simulink model "w2project2"  (R2020b)
settings: Solver=VariableStepAuto  StartTime=0.0  StopTime=10.0  RelTol=1e-3
model workspace (MAT data in the model file):
  Ie = 1
  Iv = 5
  R = 1
  be = 2
  bv = 1
  uk = 1
  us = 1.5
settings Model: Creator=rutvi  LastModifiedBy=rutvi

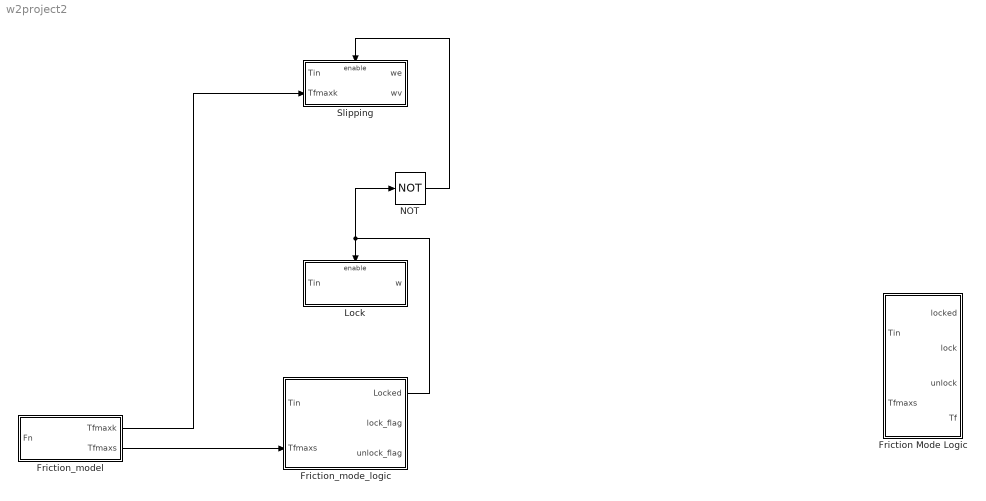
== system w2project2 ==
  Friction Mode Logic : Subsystem
      mask Display: plot([-3 1 1 3 -1 -1],[-1 -1 1 1 1 -1],-4,-5,4,5)
  Friction_mode_logic : Subsystem
  Friction_model : Subsystem
  Lock : Subsystem
  NOT : Logic  Operator=NOT  IconShape=distinctive  AllPortsSameDT=off  OutDataTypeStr=boolean
  Slipping : Subsystem
  wires:
  Friction_model/2(Tfmaxs) -> Friction_mode_logic/2(Tfmaxs)
  Friction_model/1(Tfmaxk) -> Slipping/2(Tfmaxk)
  Friction_mode_logic/1(Locked) -> NOT/1, Lock/Enable
  NOT/1 -> Slipping/Enable

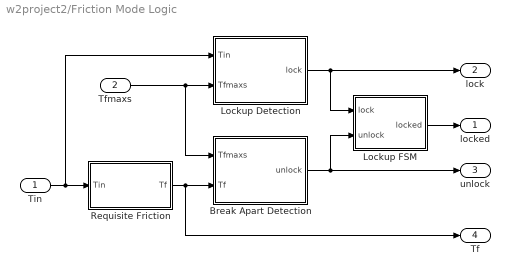
== system w2project2/Friction Mode Logic ==
  Tin : Inport
  Tfmaxs : Inport  Port=2
  Break Apart Detection : Subsystem
  Lockup Detection : Subsystem
  Lockup FSM : Subsystem
  Requisite Friction : Subsystem
  locked : Outport  InitialOutput=0  VectorParamsAs1DForOutWhenUnconnected=off
  lock : Outport  Port=2  InitialOutput=0  VectorParamsAs1DForOutWhenUnconnected=off
  unlock : Outport  Port=3  InitialOutput=0  VectorParamsAs1DForOutWhenUnconnected=off
  Tf : Outport  Port=4  InitialOutput=0  VectorParamsAs1DForOutWhenUnconnected=off
  wires:
  Tin/1 -> Lockup Detection/1(Tin), Requisite Friction/1(Tin)
  Tfmaxs/1 -> Lockup Detection/2(Tfmaxs), Break Apart Detection/1(Tfmaxs)
  Requisite Friction/1(Tf) -> Break Apart Detection/2(Tf), Tf/1
  Break Apart Detection/1(unlock) -> Lockup FSM/2(unlock), unlock/1
  Lockup Detection/1(lock) -> Lockup FSM/1(lock), lock/1
  Lockup FSM/1(locked) -> locked/1

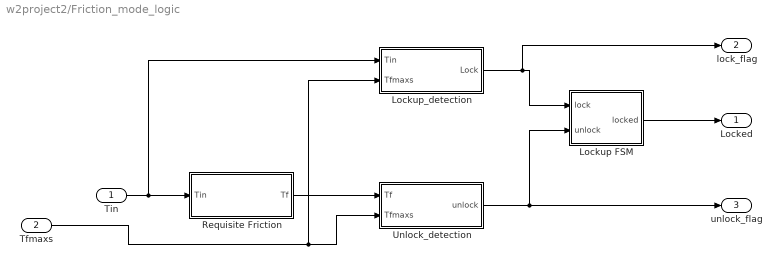
== system w2project2/Friction_mode_logic ==
  Tin : Inport
  Tfmaxs : Inport  Port=2
  Lockup FSM : Subsystem
  Lockup_detection : Subsystem
  Requisite Friction : Subsystem
  Unlock_detection : Subsystem
  Locked : Outport
  lock_flag : Outport  Port=2
  unlock_flag : Outport  Port=3
  wires:
  Lockup_detection/1(Lock) -> lock_flag/1, Lockup FSM/1(lock)
  Unlock_detection/1(unlock) -> unlock_flag/1, Lockup FSM/2(unlock)
  Lockup FSM/1(locked) -> Locked/1
  Requisite Friction/1(Tf) -> Unlock_detection/1(Tf)
  Tfmaxs/1 -> Lockup_detection/2(Tfmaxs), Unlock_detection/2(Tfmaxs)
  Tin/1 -> Lockup_detection/1(Tin), Requisite Friction/1(Tin)

== system w2project2/Friction_model ==
  Fn : Inport
  Gain : Gain  Gain=0.66*R*us
  Gain1 : Gain  Gain=0.66*R*uk
  Tfmaxk : Outport
  Tfmaxs : Outport  Port=2
  wires:
  Gain1/1 -> Tfmaxk/1
  Gain/1 -> Tfmaxs/1
  Fn/1 -> Gain1/1, Gain/1

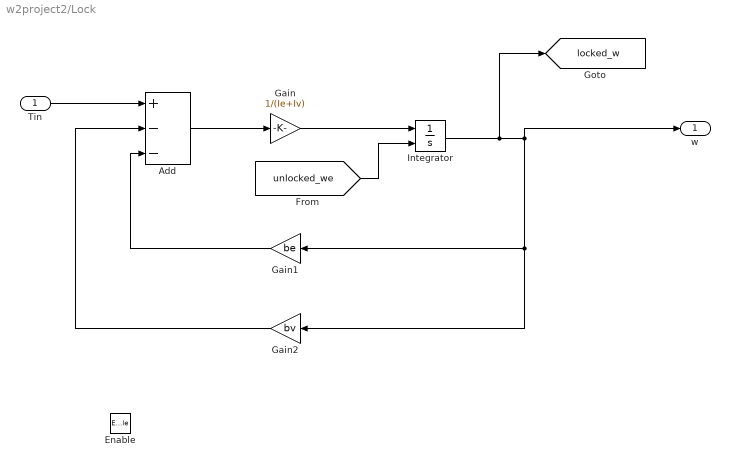
== system w2project2/Lock ==
  Tin : Inport
  Enable : EnablePort
  Add : Sum  Inputs=+--
  Gain : Gain  Gain=1/(Ie+Iv)
  Gain1 : Gain  Gain=be
  Gain2 : Gain  Gain=bv
  Integrator : Integrator  InitialConditionSource=external
  w : Outport
  tag scope: locked_w=global
  wires:
  Tin/1 -> Add/1
  Add/1 -> Gain/1
  Gain/1 -> Integrator/1
  Gain2/1 -> Add/2
  Gain1/1 -> Add/3
  [unlocked_we] -> Integrator/2
  Integrator/1 -> [locked_w], w/1, Gain2/1, Gain1/1

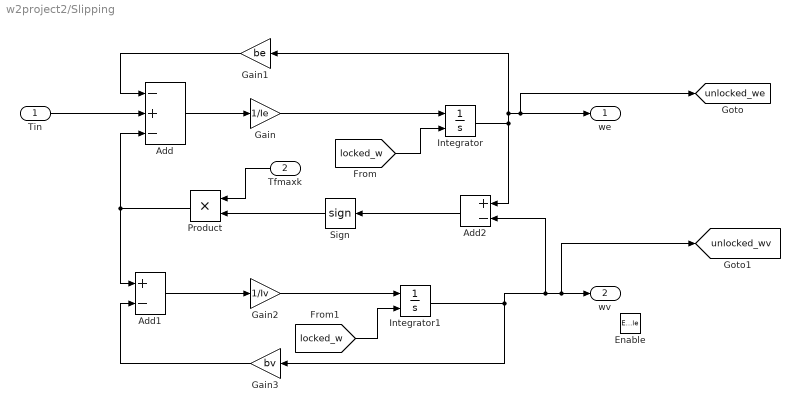
== system w2project2/Slipping ==
  Tin : Inport
  Tfmaxk : Inport  Port=2
  Enable : EnablePort
  Add : Sum  Inputs=-+-
  Add1 : Sum  Inputs=+-
  Add2 : Sum  Inputs=+-
  Gain : Gain  Gain=1/Ie
  Gain1 : Gain  Gain=be
  Gain2 : Gain  Gain=1/Iv
  Gain3 : Gain  Gain=bv
  Integrator : Integrator  InitialConditionSource=external
  Integrator1 : Integrator  InitialConditionSource=external
  Product : Product
  Sign : Signum
  we : Outport
  wv : Outport  Port=2
  tag scope: unlocked_we=global, unlocked_wv=global
  wires:
  Tin/1 -> Add/2
  Add/1 -> Gain/1
  Gain/1 -> Integrator/1
  Integrator/1 -> Gain1/1, [unlocked_we], we/1, Add2/1
  Gain1/1 -> Add/1
  Gain2/1 -> Integrator1/1
  Add1/1 -> Gain2/1
  Gain3/1 -> Add1/2
  Integrator1/1 -> Add2/2, [unlocked_wv], wv/1, Gain3/1
  Add2/1 -> Sign/1
  Sign/1 -> Product/2
  Tfmaxk/1 -> Product/1
  Product/1 -> Add1/1, Add/3
  [locked_w] -> Integrator/2
  [locked_w] -> Integrator1/2

== system w2project2/Friction Mode Logic/Break Apart Detection ==
  Tfmaxs : Inport
  Tf : Inport  Port=2
  Abs : Abs  SaturateOnIntegerOverflow=on
  Relational Operator : RelationalOperator  OutDataTypeStr=boolean  RndMeth=Nearest  InputSameDT=on
  unlock : Outport  InitialOutput=0  VectorParamsAs1DForOutWhenUnconnected=off
  wires:
  Tf/1 -> Abs/1
  Relational Operator/1 -> unlock/1
  Abs/1 -> Relational Operator/1
  Tfmaxs/1 -> Relational Operator/2

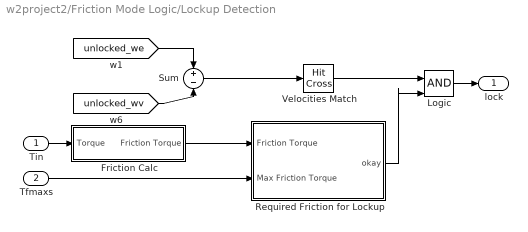
== system w2project2/Friction Mode Logic/Lockup Detection ==
  Tin : Inport
  Tfmaxs : Inport  Port=2
  Friction Calc : Subsystem
  Logic : Logic  IconShape=distinctive  OutDataTypeStr=boolean
  Required Friction for Lockup : Subsystem
  Sum : Sum  Inputs=+-  InputSameDT=on  SaturateOnIntegerOverflow=on  OutDataTypeStr=Inherit: Same as first input
  Velocities Match : HitCross
  lock : Outport  InitialOutput=0  VectorParamsAs1DForOutWhenUnconnected=off
  wires:
  Friction Calc/1(Friction Torque) -> Required Friction for Lockup/1(Friction Torque)
  Tfmaxs/1 -> Required Friction for Lockup/2(Max Friction Torque)
  Velocities Match/1 -> Logic/1
  Logic/1 -> lock/1
  Required Friction for Lockup/1(okay) -> Logic/2
  [unlocked_we] -> Sum/1
  [unlocked_wv] -> Sum/2
  Sum/1 -> Velocities Match/1
  Tin/1 -> Friction Calc/1(Torque)

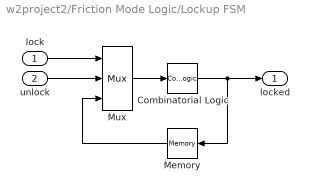
== system w2project2/Friction Mode Logic/Lockup FSM ==
  lock : Inport
  unlock : Inport  Port=2
  Combinatorial Logic : CombinatorialLogic  TruthTable=[0;1;0;0;1;1;1;0]
  Memory : Memory
  Mux : Mux  Inputs=3
  locked : Outport  InitialOutput=0  VectorParamsAs1DForOutWhenUnconnected=off
  wires:
  Memory/1 -> Mux/3
  Combinatorial Logic/1 -> locked/1, Memory/1
  unlock/1 -> Mux/2
  lock/1 -> Mux/1
  Mux/1 -> Combinatorial Logic/1

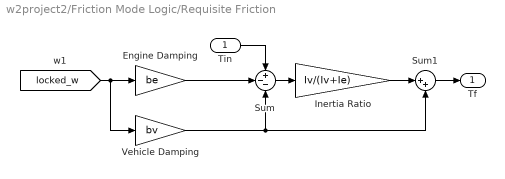
== system w2project2/Friction Mode Logic/Requisite Friction ==
  Tin : Inport
  Engine Damping : Gain  Gain=be  SaturateOnIntegerOverflow=on  OutDataTypeStr=Inherit: Same as input  ParamDataTypeStr=Inherit: Same as input
  Inertia Ratio : Gain  Gain=Iv/(Iv+Ie)  SaturateOnIntegerOverflow=on  OutDataTypeStr=Inherit: Same as input  ParamDataTypeStr=Inherit: Same as input
  Sum : Sum  Inputs=+--  InputSameDT=on  SaturateOnIntegerOverflow=on  OutDataTypeStr=Inherit: Same as first input
  Sum1 : Sum  Inputs=|++  InputSameDT=on  SaturateOnIntegerOverflow=on  OutDataTypeStr=Inherit: Same as first input
  Vehicle Damping : Gain  Gain=bv  SaturateOnIntegerOverflow=on  OutDataTypeStr=Inherit: Same as input  ParamDataTypeStr=Inherit: Same as input
  Tf : Outport  InitialOutput=0  VectorParamsAs1DForOutWhenUnconnected=off
  wires:
  [locked_w] -> Vehicle Damping/1, Engine Damping/1
  Engine Damping/1 -> Sum/2
  Vehicle Damping/1 -> Sum/3, Sum1/2
  Sum/1 -> Inertia Ratio/1
  Tin/1 -> Sum/1
  Inertia Ratio/1 -> Sum1/1
  Sum1/1 -> Tf/1

== system w2project2/Friction_mode_logic/Lockup FSM ==
  lock : Inport
  unlock : Inport  Port=2
  Combinatorial Logic : CombinatorialLogic  TruthTable=[0;1;0;0;1;1;1;0]
  Memory : Memory
  Mux : Mux  Inputs=3
  locked : Outport  InitialOutput=0  VectorParamsAs1DForOutWhenUnconnected=off
  wires:
  Memory/1 -> Mux/3
  Combinatorial Logic/1 -> locked/1, Memory/1
  unlock/1 -> Mux/2
  lock/1 -> Mux/1
  Mux/1 -> Combinatorial Logic/1

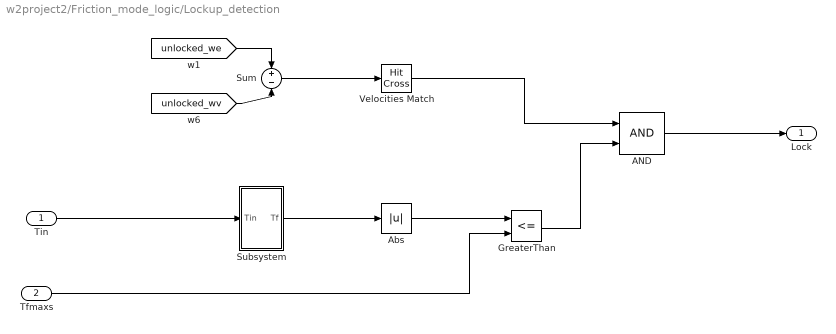
== system w2project2/Friction_mode_logic/Lockup_detection ==
  Tin : Inport
  Tfmaxs : Inport  Port=2
  AND : Logic  IconShape=distinctive  AllPortsSameDT=off  OutDataTypeStr=boolean
  Abs : Abs
  GreaterThan : RelationalOperator  Operator=<=  OutDataTypeStr=boolean  RndMeth=Simplest
  Subsystem : Subsystem
  Sum : Sum  Inputs=+-  InputSameDT=on  SaturateOnIntegerOverflow=on  OutDataTypeStr=Inherit: Same as first input
  Velocities Match : HitCross
  Lock : Outport
  wires:
  Sum/1 -> Velocities Match/1
  [unlocked_wv] -> Sum/2
  [unlocked_we] -> Sum/1
  Tin/1 -> Subsystem/1(Tin)
  Subsystem/1(Tf) -> Abs/1
  Abs/1 -> GreaterThan/1
  Tfmaxs/1 -> GreaterThan/2
  GreaterThan/1 -> AND/2
  Velocities Match/1 -> AND/1
  AND/1 -> Lock/1

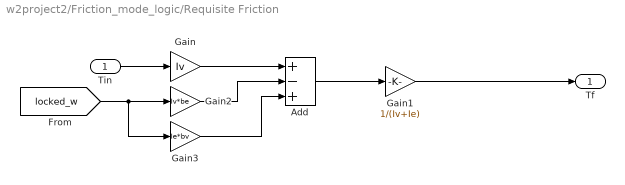
== system w2project2/Friction_mode_logic/Requisite Friction ==
  Tin : Inport
  Add : Sum  Inputs=+-+
  Gain : Gain  Gain=Iv
  Gain1 : Gain  Gain=1/(Iv+Ie)
  Gain2 : Gain  Gain=Iv*be
  Gain3 : Gain  Gain=Ie*bv
  Tf : Outport
  wires:
  Tin/1 -> Gain/1
  Gain/1 -> Add/1
  Add/1 -> Gain1/1
  Gain1/1 -> Tf/1
  Gain2/1 -> Add/2
  Gain3/1 -> Add/3
  [locked_w] -> Gain3/1, Gain2/1

== system w2project2/Friction_mode_logic/Unlock_detection ==
  Tf : Inport
  Tfmaxs : Inport  Port=2
  Abs : Abs
  GreaterThan : RelationalOperator  OutDataTypeStr=boolean  RndMeth=Simplest
  unlock : Outport
  wires:
  Tf/1 -> Abs/1
  Abs/1 -> GreaterThan/1
  Tfmaxs/1 -> GreaterThan/2
  GreaterThan/1 -> unlock/1

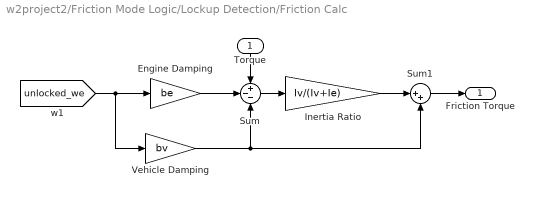
== system w2project2/Friction Mode Logic/Lockup Detection/Friction Calc ==
  Torque : Inport
  Engine Damping : Gain  Gain=be  SaturateOnIntegerOverflow=on  OutDataTypeStr=Inherit: Same as input  ParamDataTypeStr=Inherit: Same as input
  Inertia Ratio : Gain  Gain=Iv/(Iv+Ie)  SaturateOnIntegerOverflow=on  OutDataTypeStr=Inherit: Same as input  ParamDataTypeStr=Inherit: Same as input
  Sum : Sum  Inputs=+--  InputSameDT=on  SaturateOnIntegerOverflow=on  OutDataTypeStr=Inherit: Same as first input
  Sum1 : Sum  Inputs=|++  InputSameDT=on  SaturateOnIntegerOverflow=on  OutDataTypeStr=Inherit: Same as first input
  Vehicle Damping : Gain  Gain=bv  SaturateOnIntegerOverflow=on  OutDataTypeStr=Inherit: Same as input  ParamDataTypeStr=Inherit: Same as input
  Friction Torque : Outport  InitialOutput=0  VectorParamsAs1DForOutWhenUnconnected=off
  wires:
  [unlocked_we] -> Engine Damping/1, Vehicle Damping/1
  Vehicle Damping/1 -> Sum1/2, Sum/3
  Engine Damping/1 -> Sum/2
  Sum/1 -> Inertia Ratio/1
  Torque/1 -> Sum/1
  Inertia Ratio/1 -> Sum1/1
  Sum1/1 -> Friction Torque/1

== system w2project2/Friction Mode Logic/Lockup Detection/Required Friction for Lockup ==
  Friction Torque : Inport
  Max Friction Torque : Inport  Port=2
  Abs : Abs  SaturateOnIntegerOverflow=on
  Relational Operator : RelationalOperator  Operator=<=  OutDataTypeStr=boolean  RndMeth=Nearest  InputSameDT=on
  okay : Outport  InitialOutput=0  VectorParamsAs1DForOutWhenUnconnected=off
  wires:
  Friction Torque/1 -> Abs/1
  Relational Operator/1 -> okay/1
  Abs/1 -> Relational Operator/1
  Max Friction Torque/1 -> Relational Operator/2

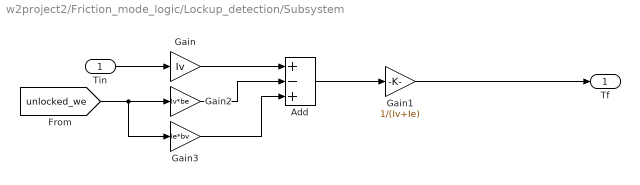
== system w2project2/Friction_mode_logic/Lockup_detection/Subsystem ==
  Tin : Inport
  Add : Sum  Inputs=+-+
  Gain : Gain  Gain=Iv
  Gain1 : Gain  Gain=1/(Iv+Ie)
  Gain2 : Gain  Gain=Iv*be
  Gain3 : Gain  Gain=Ie*bv
  Tf : Outport
  wires:
  [unlocked_we] -> Gain3/1, Gain2/1
  Gain2/1 -> Add/2
  Gain/1 -> Add/1
  Gain3/1 -> Add/3
  Gain1/1 -> Tf/1
  Tin/1 -> Gain/1
  Add/1 -> Gain1/1
